simulink model "Taller1_IdentificacionGraficaDeSistemas"  (R2024a)
settings: Solver=VariableStepAuto  StartTime=0.0  StopTime=10  RelTol=1e-3
values from neighbouring files (symbols this model uses):
  ex_sgn = datos.ex_signal_u_    [Taller1_IdentificacionGraficasDeSistemas.m]
  tau1 = respuesta(i_max) - theta    [Taller1_IdentificacionGraficasDeSistemas.m]
  theta = tiempo(find(diff(ex_sgn) ~= 0) + 1)    [Taller1_IdentificacionGraficasDeSistemas.m]
settings Model: Creator=emili  LastModifiedBy=emili

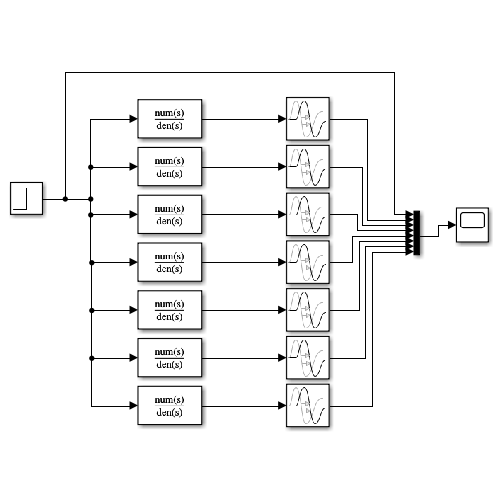
[thumbnail: Simulink's stored preview of the top-level diagram]
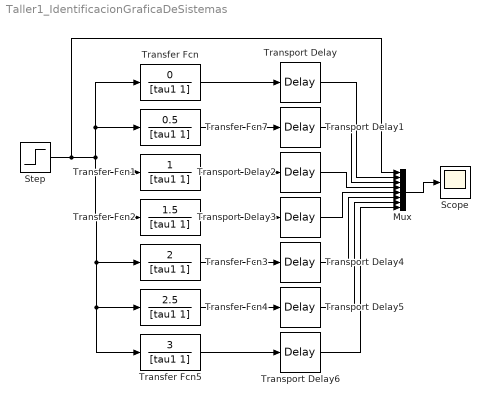
== system Taller1_IdentificacionGraficaDeSistemas ==
  Mux : Mux  Inputs=8
  Scope : Scope
  Step : Step  After=max(ex_sgn)  SampleTime=0
  Transfer Fcn : TransferFcn  Numerator=0  Denominator=[tau1 1]
  Transfer Fcn1 : TransferFcn  Numerator=1  Denominator=[tau1 1]
  Transfer Fcn2 : TransferFcn  Numerator=1.5  Denominator=[tau1 1]
  Transfer Fcn3 : TransferFcn  Numerator=2  Denominator=[tau1 1]
  Transfer Fcn4 : TransferFcn  Numerator=2.5  Denominator=[tau1 1]
  Transfer Fcn5 : TransferFcn  Numerator=3  Denominator=[tau1 1]
  Transfer Fcn7 : TransferFcn  Numerator=0.5  Denominator=[tau1 1]
  Transport Delay{,1..6} (7 alike) : TransportDelay  DelayTime=theta
  wires:
  Mux/1 -> Scope/1
  Step/1 -> Mux/1, Transfer Fcn7/1, Transfer Fcn/1, Transfer Fcn1/1, Transfer Fcn2/1, Transfer Fcn3/1, Transfer Fcn5/1, Transfer Fcn4/1
  Transfer Fcn/1 -> Transport Delay/1
  Transfer Fcn7/1 -> Transport Delay1/1
  Transfer Fcn1/1 -> Transport Delay2/1
  Transport Delay/1 -> Mux/2
  Transport Delay1/1 -> Mux/3
  Transport Delay2/1 -> Mux/4
  Transfer Fcn2/1 -> Transport Delay3/1
  Transfer Fcn3/1 -> Transport Delay4/1
  Transfer Fcn4/1 -> Transport Delay5/1
  Transport Delay3/1 -> Mux/5
  Transport Delay4/1 -> Mux/6
  Transport Delay5/1 -> Mux/7
  Transport Delay6/1 -> Mux/8
  Transfer Fcn5/1 -> Transport Delay6/1
